simulink subsystem "HardwareOutputs"  (R2019b)
settings: Solver=VariableStepAuto  StartTime=0.0  StopTime=10.0  RelTol=1e-3
undefined symbols (not defined in the file): __PRM__SERIALIZED__DATA__, SubsystemReferenceBlock
settings Model: Creator=Nick  LastModifiedBy=Nick

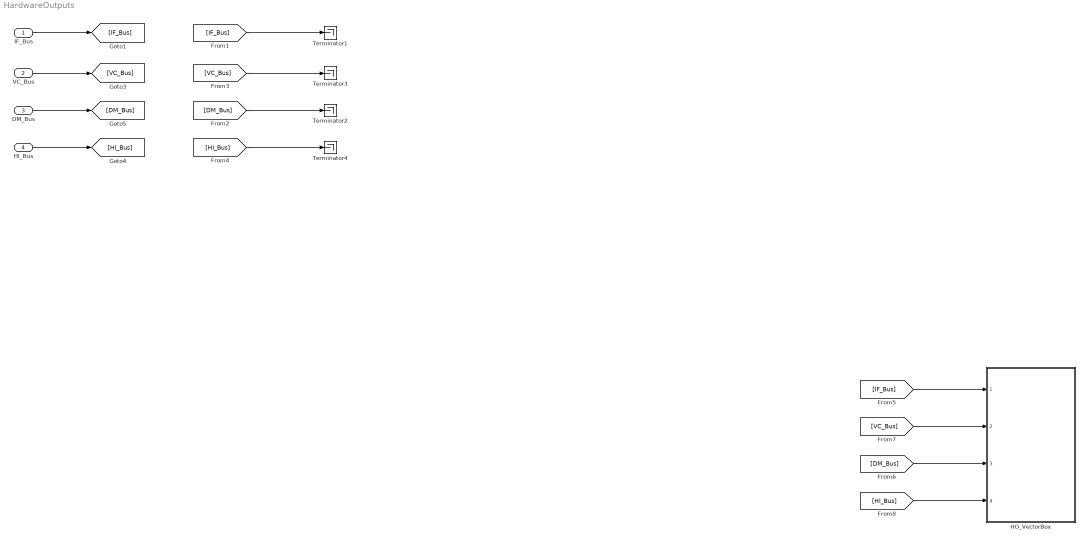
== system HardwareOutputs ==
  IF_Bus : Inport
  VC_Bus : Inport  Port=2
  DM_Bus : Inport  Port=3
  HI_Bus : Inport  Port=4
  HO_VectorBox : Subsystem  BlockKeywords=__PRM__SERIALIZED__DATA__:SubsystemReferenceBlock  ReferencedSubsystem=HO_VectorBox
  Terminator{1..4} (4 alike) : Terminator
  wires:
  [VC_Bus] -> Terminator3/1
  VC_Bus/1 -> [VC_Bus]
  [IF_Bus] -> Terminator1/1
  HI_Bus/1 -> [HI_Bus]
  [HI_Bus] -> Terminator4/1
  IF_Bus/1 -> [IF_Bus]
  DM_Bus/1 -> [DM_Bus]
  [DM_Bus] -> Terminator2/1
  [IF_Bus] -> HO_VectorBox/1
  [DM_Bus] -> HO_VectorBox/3
  [HI_Bus] -> HO_VectorBox/4
  [VC_Bus] -> HO_VectorBox/2
